simulink model "PACEWIPgbug2version13"  (R2022b)
settings: Solver=FixedStepAuto  StartTime=0.0  StopTime=10  FixedStep=1e-3  RelTol=1e-3  EnableMultiTasking=on
undefined symbols (not defined in the file): A0, A1, D0, D1, D10, D11, D12, D13, D2, D3, D4, D5, D6, D7, D8, D9, PTA0, PTA1, PTA2, PTB2, PTB23, PTB3, PTB9, PTC16, PTC17, PTC2, PTC3, PTC4, PTD0, PTD1, PTD2, PTD3
libraries: frdmk64flib x21
settings Model: PacingRate=0.400000  ExtModeTrigDuration=5  Creator=carlo  LastModifiedBy=skaad
settings OptimizationCC: EnhancedBackFolding=on  PassReuseOutputArgsThreshold=0  MaxStackSize=64  OptimizeBlockOrder=speed  DifferentSizesBufferReuse=on  OptimizationCustomize=off
settings DebuggingCC: ParameterTunabilityLossMsg=error  UnconnectedInputMsg=warning  UnconnectedOutputMsg=warning  UnconnectedLineMsg=warning
settings HardwareCC: ProdBitPerPointer=32  ProdBitPerSizeT=32  ProdBitPerPtrDiffT=32  ProdLargestAtomicInteger=Long  ProdLargestAtomicFloat=Double  ProdWordSize=32  ProdHWDeviceType=ARM Compatible->ARM Cortex  UseEmbeddedCoderFeatures=off
settings ModelReferenceCC: EnableRefExpFcnMdlSchedulingChecks=on
settings SFSimCC: MATLABDynamicMemAlloc=off
settings RTWCC: Description=Embedded Coder  SystemTargetFile=ert.tlc  HardwareBoard=NXP FRDM-K64F  TLCOptions="-aInlineSetEventsForThisBaseRateFcn=TLC_FALSE -aSuppressMultiTaskScheduler=TLC_FALSE  -aRateBasedStepFcn=0"  TemplateMakefile=ert_default_tmf  Toolchain=GNU Tools for ARM Embedded Processors  DLArmComputeVersion=19.05
settings CodeAppCC: ForceParamTrailComments=on  OperatorAnnotations=on
settings ERTTargetCC: ERTCustomFileBanners=off  SupportContinuousTime=on  SupportNonInlinedSFcns=on  RemoveResetFunc=off  ModelStepFunctionPrototypeControlCompliant=off  ExtModeTransport=4  ExtModeMexFile=sendToCommService

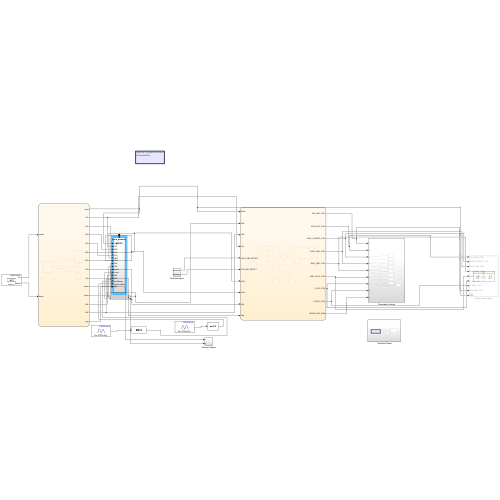
[thumbnail: Simulink's stored preview of the top-level diagram]
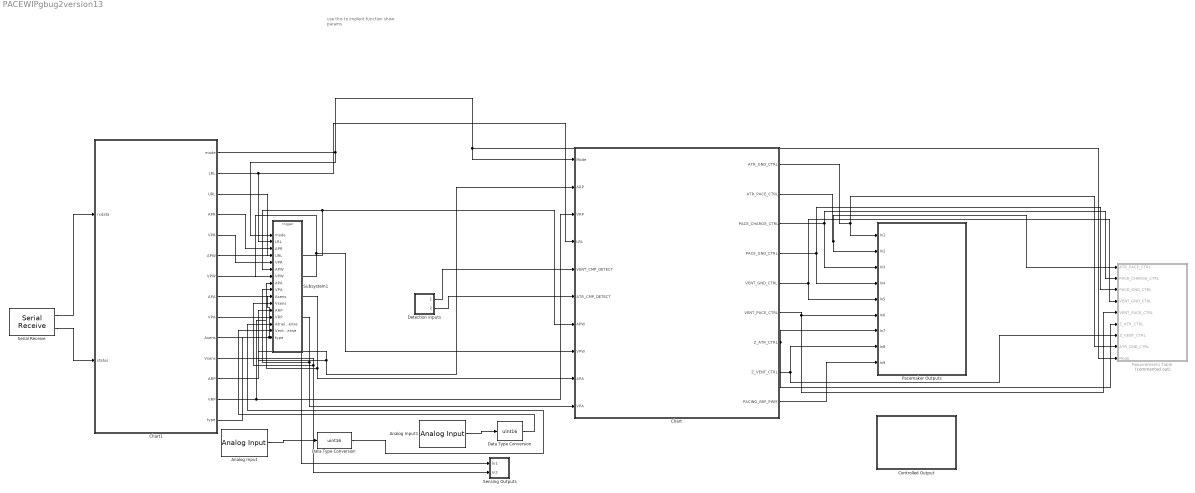
== system PACEWIPgbug2version13 ==
  note: use this to implent function
      | show params
  Analog Input : frdmk64flib/Analog Input  Whichpin=PTB2 (A0)  SampleTime=-1
  Analog Input1 : frdmk64flib/Analog Input  Whichpin=PTB3 (A1)  SampleTime=-1
  Chart : Stateflow chart  TreatAsAtomicUnit=on
  Chart1 : Stateflow chart  TreatAsAtomicUnit=on
  Controlled Output : Subsystem
  Data Type Conversion : DataTypeConversion  OutDataTypeStr=uint16  SaturateOnIntegerOverflow=off  RndMeth=Floor
  Data Type Conversion : DataTypeConversion  OutDataTypeStr=uint16  SaturateOnIntegerOverflow=off  RndMeth=Floor
  Detection inputs : Subsystem
  Pacemaker Outputs : Subsystem
  Requirements Table : Requirements Table  Commented=on  TreatAsAtomicUnit=on
  Sensing Outputs : Subsystem
  Serial Receive : frdmk64flib/Serial Receive  SCIModule=0  Baudrate=uint32(9600)  Parity=None  StopBits=1  HardwareFlowControl=None  ByteOrder=LittleEndian  DataType=uint8  DataLength=28  BlockingMode=off  OutputStatus=on  SampleTime=-1
  Subsystem1 : Subsystem
  wires:
  Chart/1(ATR_GND_CTRL) -> Requirements Table/8(ATR_GND_CTRL), Pacemaker Outputs/1(In1)
  Chart/2(ATR_PACE_CTRL) -> Requirements Table/1(ATR_PACE_CTRL), Pacemaker Outputs/2(In2)
  Chart/4(PACE_GND_CTRL) -> Pacemaker Outputs/4(In4), Requirements Table/3(PACE_GND_CTRL)
  Chart/5(VENT_GND_CTRL) -> Pacemaker Outputs/5(In5), Requirements Table/4(VENT_GND_CTRL)
  Chart/6(VENT_PACE_CTRL) -> Requirements Table/5(VENT_PACE_CTRL), Pacemaker Outputs/6(In6)
  Chart/7(Z_ATR_CTRL) -> Requirements Table/6(Z_ATR_CTRL), Pacemaker Outputs/7(In7)
  Chart/8(Z_VENT_CTRL) -> Requirements Table/7(Z_VENT_CTRL), Pacemaker Outputs/8(In8)
  Chart/9(PACING_REF_PWM) -> Pacemaker Outputs/9(In9)
  Chart/3(PACE_CHARGE_CTRL) -> Pacemaker Outputs/3(In3), Requirements Table/2(PACE_CHARGE_CTRL)
  Chart1/1(mode) -> Chart/1(Mode), Requirements Table/9(Mode), Subsystem1/1(mode)
  Chart1/12(ARP) -> Chart/2(ARP), Subsystem1/12(ARP)
  Chart1/13(VRP) -> Chart/3(VRP), Subsystem1/13(VRP)
  Chart1/2(LRL) -> Chart/4(LRL), Subsystem1/2(LRL)
  Chart1/6(APW) -> Chart/7(APW), Subsystem1/6(APW)
  Serial Receive/1 -> Chart1/1(rxdata)
  Chart1/3(URL) -> Subsystem1/4(URL)
  Chart1/4(APR) -> Subsystem1/3(APR)
  Chart1/5(VPR) -> Subsystem1/5(VPR)
  Chart1/7(VPW) -> Subsystem1/7(VPW), Chart/8(VPW)
  Chart1/8(APA) -> Subsystem1/8(APA), Chart/9(APA)
  Chart1/9(VPA) -> Subsystem1/9(VPA), Chart/10(VPA)
  Detection inputs/1(VentricularSense) -> Chart/5(VENT_CMP_DETECT)
  Detection inputs/2(AtrialSense) -> Chart/6(ATR_CMP_DETECT)
  Chart1/11(Vsens) -> Subsystem1/11(Vsens), Sensing Outputs/2(In2)
  Chart1/10(Asens) -> Sensing Outputs/1(In1), Subsystem1/10(Asens)
  Serial Receive/2 -> Chart1/2(status)
  Analog Input1/1 -> Data Type Conversion/1
  Data Type Conversion/1 -> Subsystem1/15(VentricularSense)
  Analog Input/1 -> Data Type Conversion/1
  Data Type Conversion/1 -> Subsystem1/14(AtrialSense)
  Chart1/14(type) -> Subsystem1/16(type)

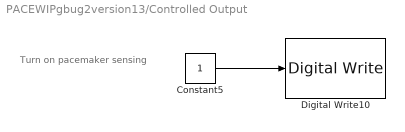
== system PACEWIPgbug2version13/Controlled Output ==
  note: Turn on pacemaker
      | sensing
  Constant5 : Constant
  Digital Write10 : frdmk64flib/Digital Write  Whichpin=PTD1 (D13)
  wires:
  Constant5/1 -> Digital Write10/1

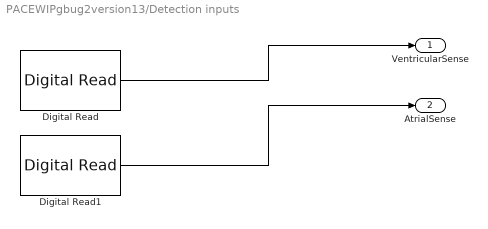
== system PACEWIPgbug2version13/Detection inputs ==
  Digital Read : frdmk64flib/Digital Read  Whichpin=PTC17 (D1)  SampleTime=-1
  Digital Read1 : frdmk64flib/Digital Read  Whichpin=PTC16 (D0)  SampleTime=-1
  VentricularSense : Outport
  AtrialSense : Outport  Port=2
  wires:
  Digital Read/1 -> VentricularSense/1
  Digital Read1/1 -> AtrialSense/1

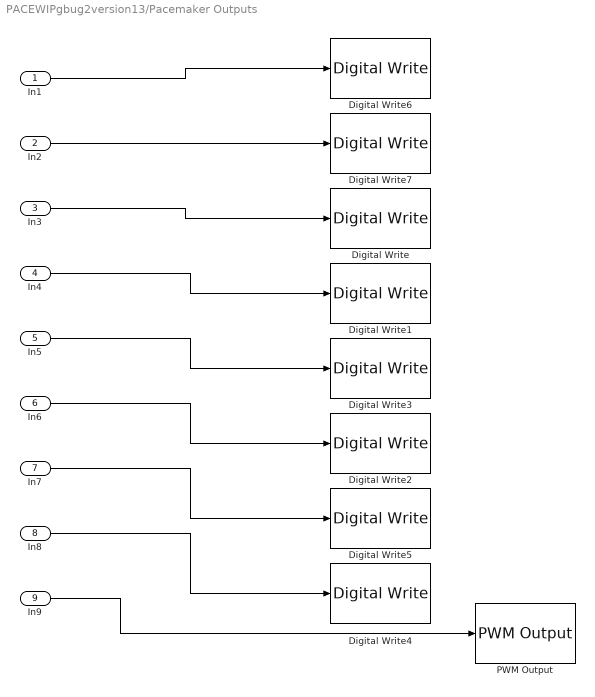
== system PACEWIPgbug2version13/Pacemaker Outputs ==
  In1 : Inport
  In2 : Inport  Port=2
  In3 : Inport  Port=3
  In4 : Inport  Port=4
  In5 : Inport  Port=5
  In6 : Inport  Port=6
  In7 : Inport  Port=7
  In8 : Inport  Port=8
  In9 : Inport  Port=9
  Digital Write : frdmk64flib/Digital Write  Whichpin=PTB9 (D2)
  Digital Write1 : frdmk64flib/Digital Write  Whichpin=PTD0 (D10)
  Digital Write2 : frdmk64flib/Digital Write  Whichpin=PTC4 (D9)
  Digital Write3 : frdmk64flib/Digital Write  Whichpin=PTD3 (D12)
  Digital Write4 : frdmk64flib/Digital Write  Whichpin=PTC3 (D7)
  Digital Write5 : frdmk64flib/Digital Write  Whichpin=PTB23 (D4)
  Digital Write6 : frdmk64flib/Digital Write  Whichpin=PTD2 (D11)
  Digital Write7 : frdmk64flib/Digital Write  Whichpin=PTA0 (D8)
  PWM Output : frdmk64flib/PWM Output  Whichpin=PTA2 (D5)  InitialFrequency=2000  InitialDutyCycle=60
  wires:
  In1/1 -> Digital Write6/1
  In3/1 -> Digital Write/1
  In2/1 -> Digital Write7/1
  In4/1 -> Digital Write1/1
  In9/1 -> PWM Output/1
  In7/1 -> Digital Write5/1
  In6/1 -> Digital Write2/1
  In8/1 -> Digital Write4/1
  In5/1 -> Digital Write3/1

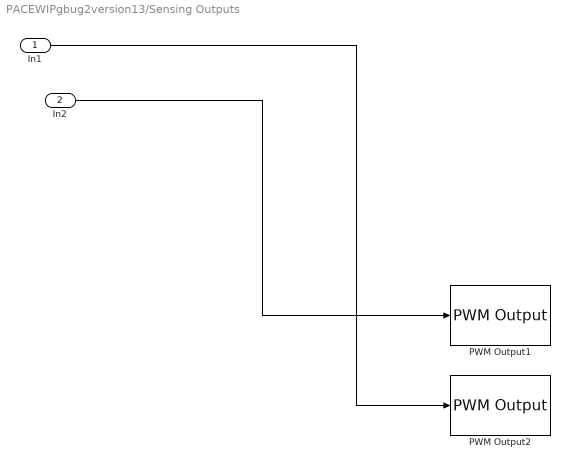
== system PACEWIPgbug2version13/Sensing Outputs ==
  In1 : Inport
  In2 : Inport  Port=2
  PWM Output1 : frdmk64flib/PWM Output  Whichpin=PTA1 (D3)  InitialFrequency=2000  InitialDutyCycle=60
  PWM Output2 : frdmk64flib/PWM Output  Whichpin=PTC2 (D6)  InitialFrequency=2000  InitialDutyCycle=60
  wires:
  In1/1 -> PWM Output2/1
  In2/1 -> PWM Output1/1

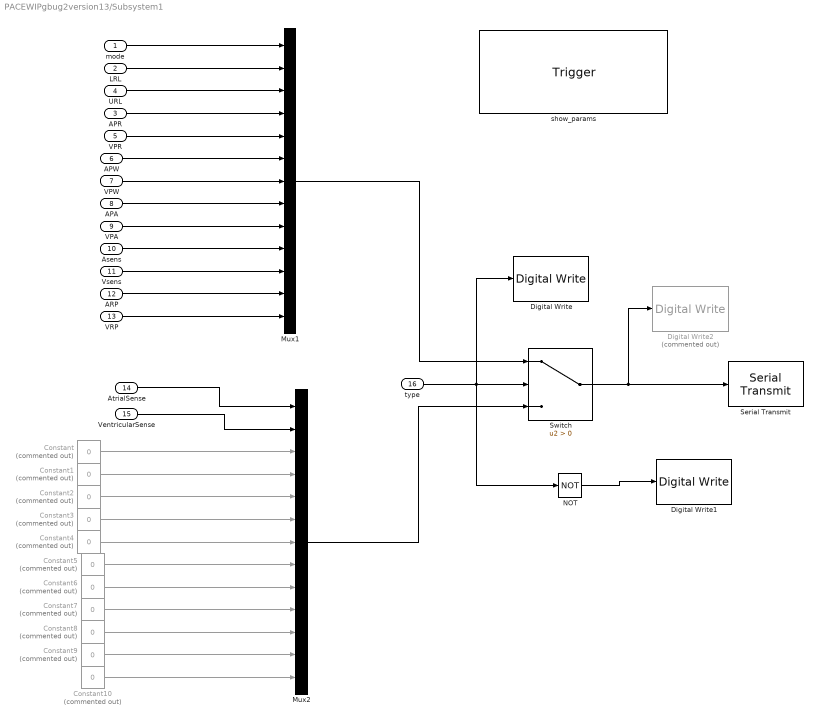
== system PACEWIPgbug2version13/Subsystem1 ==
  mode : Inport
  LRL : Inport  Port=2
  APR : Inport  Port=3
  URL : Inport  Port=4
  VPR : Inport  Port=5
  APW : Inport  Port=6
  VPW : Inport  Port=7
  APA : Inport  Port=8
  VPA : Inport  Port=9
  Asens : Inport  Port=10
  Vsens : Inport  Port=11
  ARP : Inport  Port=12
  VRP : Inport  Port=13
  AtrialSense : Inport  Port=14
  VentricularSense : Inport  Port=15
  type : Inport  Port=16
  show_params : TriggerPort  TriggerType=function-call  IsSimulinkFunction=on  FunctionName=show_params  VariantControl=(inherit)
  Constant{,1..10} (11 alike) : Constant  Commented=on  Value=0  OutDataTypeStr=uint16
  Digital Write : frdmk64flib/Digital Write  Whichpin=BLUE_LED
  Digital Write1 : frdmk64flib/Digital Write  Whichpin=RED_LED
  Digital Write2 : frdmk64flib/Digital Write  Commented=on  Whichpin=GREEN_LED
  Mux1 : Mux  Inputs=13
  Mux2 : Mux  Inputs=13
  NOT : Logic  Operator=NOT  IconShape=distinctive  AllPortsSameDT=off  OutDataTypeStr=boolean
  Serial Transmit : frdmk64flib/Serial Transmit  SCIModule=0  Baudrate=uint32(9600)  Parity=None  StopBits=1  HardwareFlowControl=None  ByteOrder=LittleEndian  BlockingMode=on  OutputStatus=off
  Switch : Switch  Criteria=u2 > Threshold  SaturateOnIntegerOverflow=off  InputSameDT=off
  wires:
  VPR/1 -> Mux1/5
  VPA/1 -> Mux1/9
  ARP/1 -> Mux1/12
  APA/1 -> Mux1/8
  mode/1 -> Mux1/1
  Asens/1 -> Mux1/10
  VPW/1 -> Mux1/7
  APR/1 -> Mux1/4
  LRL/1 -> Mux1/2
  VRP/1 -> Mux1/13
  Vsens/1 -> Mux1/11
  Mux1/1 -> Switch/1
  type/1 -> NOT/1, Digital Write/1, Switch/2
  APW/1 -> Mux1/6
  URL/1 -> Mux1/3
  Switch/1 -> Digital Write2/1, Serial Transmit/1
  Constant/1 -> Mux2/3
  Constant1/1 -> Mux2/4
  AtrialSense/1 -> Mux2/1
  VentricularSense/1 -> Mux2/2
  Constant2/1 -> Mux2/5
  Constant3/1 -> Mux2/6
  Constant6/1 -> Mux2/9
  Constant7/1 -> Mux2/10
  Constant5/1 -> Mux2/8
  Constant4/1 -> Mux2/7
  Constant8/1 -> Mux2/11
  Constant9/1 -> Mux2/12
  Constant10/1 -> Mux2/13
  Mux2/1 -> Switch/3
  NOT/1 -> Digital Write1/1

== stateflow chart PACEWIPgbug2version13/Requirements Table ==
  (default) -> (junction 1073746513)
  (junction 1073746513) -> (junction 1073746514) : {
      | % SF_REQ_REV_07
      | }
  (junction 1073746514) -> (junction 1073746516) : {
      | % HEADER_ASSIGNMENTS
      |
      | }
  (junction 1073746516) -> (junction 1073746518) : {
      | % START_A_4
      | }
  (junction 1073746518) -> (junction 1073746520) : {
      | }
  (junction 1073746520) -> (junction 1073746522)
  (junction 1073746522) -> (junction 1073746524) : {
      | }
  (junction 1073746524) -> (junction 1073746526) : {
      | % END_A_4
      | }
  (junction 1073746526) -> (junction 1073746528) : {
      | % START_R_1
      | }
  (junction 1073746528) -> (junction 1073746530) : {
      | }
  (junction 1073746530) -> (junction 1073746532) : {
      |
      |
      | }
  (junction 1073746532) -> (junction 1073746534) : {
      | }
  (junction 1073746534) -> (junction 1073746590) : {
      | % START_R_16
      | }
  (junction 1073746590) -> (junction 1073746592) : {
      | }
  (junction 1073746592) -> (junction 1073746594)
  (junction 1073746594) -> (junction 1073746596) [order 1] : [duration((Mode==1)) >= 1]
  (junction 1073746594) -> (junction 1073746602) [order 2]
  (junction 1073746596) -> (junction 1073746598) : {
      | reqtable_postcondition((((ATR_PACE_CTRL) == (0))) && (((VENT_PACE_CTRL) == (0))) && (((PACE_CHARGE_CTRL) == (1))) && (((PACE_GND_CTRL) == (0))) && (((ATR_GND_CTRL) == (1))) && (((VENT_GND_CTRL) == (0))) && (((Z_ATR_CTRL) == (0))) && (((Z_VENT_CTRL) == (0))), 'R:1.1');
      |
      |
      | }
  (junction 1073746598) -> (junction 1073746600) : {
      | }
  (junction 1073746600) -> (junction 1073746602)
  (junction 1073746602) -> (junction 1073746604)
  (junction 1073746604) -> (junction 1073746606) : {
      | % END_R_16
      | }
  (junction 1073746606) -> (junction 1073746611) : {
      | % START_R_22
      | }
  (junction 1073746611) -> (junction 1073746613) : {
      | }
  (junction 1073746613) -> (junction 1073746615)
  (junction 1073746615) -> (junction 1073746617) [order 1] : [duration((Mode==1)) >= 1]
  (junction 1073746615) -> (junction 1073746623) [order 2]
  (junction 1073746617) -> (junction 1073746619) : {
      | reqtable_postcondition((((ATR_PACE_CTRL) == (1))) && (((VENT_PACE_CTRL) == (0))) && (((PACE_CHARGE_CTRL) == (0))) && (((PACE_GND_CTRL) == (1))) && (((ATR_GND_CTRL) == (0))) && (((VENT_GND_CTRL) == (0))) && (((Z_ATR_CTRL) == (0))) && (((Z_VENT_CTRL) == (0))), 'R:1.2');
      |
      |
      | }
  (junction 1073746619) -> (junction 1073746621) : {
      | }
  (junction 1073746621) -> (junction 1073746623)
  (junction 1073746623) -> (junction 1073746625)
  (junction 1073746625) -> (junction 1073746627) : {
      | % END_R_22
      | }
  (junction 1073746627) -> (junction 1073746556) : {
      | % END_R_1
      | }
  (junction 1073746556) -> (junction 1073746674) : {
      | % START_R_7
      | }
  (junction 1073746674) -> (junction 1073746676) : {
      | }
  (junction 1073746676) -> (junction 1073746678) : {
      |
      |
      | }
  (junction 1073746678) -> (junction 1073746680) : {
      | }
  (junction 1073746680) -> (junction 1073746682) : {
      | % START_R_28
      | }
  (junction 1073746682) -> (junction 1073746684) : {
      | }
  (junction 1073746684) -> (junction 1073746686)
  (junction 1073746686) -> (junction 1073746688) [order 1] : [duration((Mode==2)) >= 1]
  (junction 1073746686) -> (junction 1073746694) [order 2]
  (junction 1073746688) -> (junction 1073746690) : {
      | reqtable_postcondition((((ATR_PACE_CTRL) == (0))) && (((VENT_PACE_CTRL) == (0))) && (((PACE_CHARGE_CTRL) == (1))) && (((PACE_GND_CTRL) == (0))) && (((ATR_GND_CTRL) == (0))) && (((VENT_GND_CTRL) == (1))) && (((Z_ATR_CTRL) == (0))) && (((Z_VENT_CTRL) == (0))), 'R:2.1');
      |
      |
      | }
  (junction 1073746690) -> (junction 1073746692) : {
      | }
  (junction 1073746692) -> (junction 1073746694)
  (junction 1073746694) -> (junction 1073746696)
  (junction 1073746696) -> (junction 1073746698) : {
      | % END_R_28
      | }
  (junction 1073746698) -> (junction 1073746700) : {
      | % START_R_31
      | }
  (junction 1073746700) -> (junction 1073746702) : {
      | }
  (junction 1073746702) -> (junction 1073746704)
  (junction 1073746704) -> (junction 1073746706) [order 1] : [duration((Mode==2)) >= 1]
  (junction 1073746704) -> (junction 1073746712) [order 2]
  (junction 1073746706) -> (junction 1073746708) : {
      | reqtable_postcondition((((ATR_PACE_CTRL) == (0))) && (((VENT_PACE_CTRL) == (1))) && (((PACE_CHARGE_CTRL) == (0))) && (((PACE_GND_CTRL) == (1))) && (((ATR_GND_CTRL) == (0))) && (((VENT_GND_CTRL) == (0))) && (((Z_ATR_CTRL) == (0))) && (((Z_VENT_CTRL) == (0))), 'R:2.2');
      |
      |
      | }
  (junction 1073746708) -> (junction 1073746710) : {
      | }
  (junction 1073746710) -> (junction 1073746712)
  (junction 1073746712) -> (junction 1073746714)
  (junction 1073746714) -> (junction 1073746716) : {
      | % END_R_31
      | }
  (junction 1073746716) -> (junction 1073746718) : {
      | % END_R_7
      | }
  (junction 1073746718) -> (junction 1073746724) : {
      | % START_R_10
      | }
  (junction 1073746724) -> (junction 1073746726) : {
      | }
  (junction 1073746726) -> (junction 1073746728) : {
      |
      |
      | }
  (junction 1073746728) -> (junction 1073746730) : {
      | }
  (junction 1073746730) -> (junction 1073746732) : {
      | % START_R_46
      | }
  (junction 1073746732) -> (junction 1073746734) : {
      | }
  (junction 1073746734) -> (junction 1073746736)
  (junction 1073746736) -> (junction 1073746738) [order 1] : [duration((Mode==3)) >= 1]
  (junction 1073746736) -> (junction 1073746744) [order 2]
  (junction 1073746738) -> (junction 1073746740) : {
      | reqtable_postcondition((((ATR_PACE_CTRL) == (0))) && (((VENT_PACE_CTRL) == (0))) && (((PACE_CHARGE_CTRL) == (1))) && (((PACE_GND_CTRL) == (0))) && (((ATR_GND_CTRL) == (1))) && (((VENT_GND_CTRL) == (0))) && (((Z_ATR_CTRL) == (0))) && (((Z_VENT_CTRL) == (0))), 'R:3.1');
      |
      |
      | }
  (junction 1073746740) -> (junction 1073746742) : {
      | }
  (junction 1073746742) -> (junction 1073746744)
  (junction 1073746744) -> (junction 1073746746)
  (junction 1073746746) -> (junction 1073746748) : {
      | % END_R_46
      | }
  (junction 1073746748) -> (junction 1073746750) : {
      | % START_R_61
      | }
  (junction 1073746750) -> (junction 1073746752) : {
      | }
  (junction 1073746752) -> (junction 1073746754)
  (junction 1073746754) -> (junction 1073746756) [order 1] : [duration((Mode==3)) >= 1]
  (junction 1073746754) -> (junction 1073746762) [order 2]
  (junction 1073746756) -> (junction 1073746758) : {
      | reqtable_postcondition((((ATR_PACE_CTRL) == (1))) && (((VENT_PACE_CTRL) == (0))) && (((PACE_CHARGE_CTRL) == (0))) && (((PACE_GND_CTRL) == (1))) && (((ATR_GND_CTRL) == (0))) && (((VENT_GND_CTRL) == (0))) && (((Z_ATR_CTRL) == (0))) && (((Z_VENT_CTRL) == (0))), 'R:3.2');
      |
      |
      | }
  (junction 1073746758) -> (junction 1073746760) : {
      | }
  (junction 1073746760) -> (junction 1073746762)
  (junction 1073746762) -> (junction 1073746764)
  (junction 1073746764) -> (junction 1073746766) : {
      | % END_R_61
      | }
  (junction 1073746766) -> (junction 1073746768) : {
      | % END_R_10
      | }
  (junction 1073746768) -> (junction 1073746774) : {
      | % START_R_13
      | }
  (junction 1073746774) -> (junction 1073746776) : {
      | }
  (junction 1073746776) -> (junction 1073746778) : {
      |
      |
      | }
  (junction 1073746778) -> (junction 1073746780) : {
      | }
  (junction 1073746780) -> (junction 1073746782) : {
      | % START_R_49
      | }
  (junction 1073746782) -> (junction 1073746784) : {
      | }
  (junction 1073746784) -> (junction 1073746786)
  (junction 1073746786) -> (junction 1073746788) [order 1] : [duration((Mode==4)) >= 1]
  (junction 1073746786) -> (junction 1073746794) [order 2]
  (junction 1073746788) -> (junction 1073746790) : {
      | reqtable_postcondition((((ATR_PACE_CTRL) == (0))) && (((VENT_PACE_CTRL) == (0))) && (((PACE_CHARGE_CTRL) == (1))) && (((PACE_GND_CTRL) == (0))) && (((ATR_GND_CTRL) == (0))) && (((VENT_GND_CTRL) == (1))) && (((Z_ATR_CTRL) == (0))) && (((Z_VENT_CTRL) == (0))), 'R:4.1');
      |
      |
      | }
  (junction 1073746790) -> (junction 1073746792) : {
      | }
  (junction 1073746792) -> (junction 1073746794)
  (junction 1073746794) -> (junction 1073746796)
  (junction 1073746796) -> (junction 1073746798) : {
      | % END_R_49
      | }
  (junction 1073746798) -> (junction 1073746800) : {
      | % START_R_58
      | }
  (junction 1073746800) -> (junction 1073746802) : {
      | }
  (junction 1073746802) -> (junction 1073746804)
  (junction 1073746804) -> (junction 1073746806) [order 1] : [duration((Mode==4)) >= 1]
  (junction 1073746804) -> (junction 1073746812) [order 2]
  (junction 1073746806) -> (junction 1073746808) : {
      | reqtable_postcondition((((ATR_PACE_CTRL) == (0))) && (((VENT_PACE_CTRL) == (1))) && (((PACE_CHARGE_CTRL) == (0))) && (((PACE_GND_CTRL) == (1))) && (((ATR_GND_CTRL) == (0))) && (((VENT_GND_CTRL) == (0))) && (((Z_ATR_CTRL) == (0))) && (((Z_VENT_CTRL) == (0))), 'R:4.2');
      |
      |
      | }
  (junction 1073746808) -> (junction 1073746810) : {
      | }
  (junction 1073746810) -> (junction 1073746812)
  (junction 1073746812) -> (junction 1073746814)
  (junction 1073746814) -> (junction 1073746816) : {
      | % END_R_58
      | }
  (junction 1073746816) -> (junction 1073746818) : {
      | % END_R_13
      | }
  data: ATR_PACE_CTRL input double; PACE_CHARGE_CTRL input; PACE_GND_CTRL input; VENT_GND_CTRL input; VENT_PACE_CTRL input; Z_ATR_CTRL input; Z_VENT_CTRL input; ATR_GND_CTRL input; Mode input

== stateflow chart PACEWIPgbug2version13/Chart ==
  state AOO_PACE
    entry:
    PACE_CHARGE_CTRL=0;
    PACE_GND_CTRL=1;
    VENT_PACE_CTRL=0
    VENT_GND_CTRL=0;
    Z_ATR_CTRL=0;
    Z_VENT_CTRL=0;
    ATR_GND_CTRL=0;
    ATR_PACE_CTRL=1
  state AOO_CHARGE
    entry:
    ATR_PACE_CTRL=0;
    VENT_PACE_CTRL=0;
    PACING_REF_PWM=APA;
    PACE_CHARGE_CTRL=1;
    PACE_GND_CTRL=1;
    Z_ATR_CTRL=0;
    Z_VENT_CTRL=0;
    VENT_GND_CTRL=0;
    ATR_GND_CTRL=1
  state VVI_CHARGE
    ATR_PACE_CTRL=0;
    VENT_PACE_CTRL=0;
    PACING_REF_PWM=VPA;
    PACE_CHARGE_CTRL=1;
    PACE_GND_CTRL=1;
    Z_ATR_CTRL=0;
    Z_VENT_CTRL=0;
    ATR_GND_CTRL=0;
    VENT_GND_CTRL=1
  state VVI_Refractory
  state MODE_SELECT
  state VOO_CHARGE
    entry:
    ATR_PACE_CTRL=0;
    VENT_PACE_CTRL=0;
    PACING_REF_PWM=VPA;
    PACE_CHARGE_CTRL=1;
    PACE_GND_CTRL=1;
    Z_ATR_CTRL=0;
    Z_VENT_CTRL=0;
    ATR_GND_CTRL=0;
    VENT_GND_CTRL=1
  state VOO_PACE
    entry:
    PACE_CHARGE_CTRL=0;
    PACE_GND_CTRL=1;
    ATR_PACE_CTRL=0
    ATR_GND_CTRL=0;
    Z_ATR_CTRL=0;
    Z_VENT_CTRL=0;
    VENT_GND_CTRL=0;
    VENT_PACE_CTRL=1
  state VVI_SENSING
  state VVI_PACE
    entry:
    PACE_CHARGE_CTRL=0;
    PACE_GND_CTRL=1;
    ATR_PACE_CTRL=0
    ATR_GND_CTRL=0;
    Z_ATR_CTRL=0;
    Z_VENT_CTRL=0;
    VENT_GND_CTRL=0;
    VENT_PACE_CTRL=1
  state AAI_CHARGE
    entry:
    ATR_PACE_CTRL = 0;
    VENT_PACE_CTRL = 0;
    PACING_REF_PWM = APA;
    PACE_CHARGE_CTRL = 1;
    PACE_GND_CTRL = 1;
    Z_ATR_CTRL = 0;
    Z_VENT_CTRL = 0;
    VENT_GND_CTRL = 0;
    ATR_GND_CTRL = 1
  state AAI_Refractory
  state AAI_SENSING
  state AAI_PACE
    entry:
    PACE_CHARGE_CTRL = 0;
    PACE_GND_CTRL = 1;
    VENT_PACE_CTRL = 0;
    VENT_GND_CTRL = 0;
    Z_ATR_CTRL = 0;
    Z_VENT_CTRL = 0;
    ATR_GND_CTRL = 0;
    ATR_PACE_CTRL = 1
  MODE_SELECT -> VVI_CHARGE [order 3] : [Mode==4]
  VVI_CHARGE -> MODE_SELECT [order 1] : [Mode~=4]
  AOO_CHARGE -> AOO_PACE [order 1] : after(1000-APW,msec)
  AOO_PACE -> AOO_CHARGE : after(APW,msec)
  MODE_SELECT -> AOO_CHARGE [order 2] : [Mode == 1]
  VVI_PACE -> VVI_CHARGE : after(VPW,msec)
  (default) -> MODE_SELECT
  VVI_CHARGE -> VVI_Refractory [order 2] : after(1,msec)
  AOO_CHARGE -> MODE_SELECT [order 2] : [Mode~=1]
  VVI_SENSING -> VVI_Refractory [order 2] : [VENT_CMP_DETECT == 1]
  MODE_SELECT -> VOO_CHARGE [order 1] : [Mode == 2]
  VVI_Refractory -> VVI_SENSING : after(VRP,msec)
  VOO_CHARGE -> MODE_SELECT [order 2] : [Mode~=2]
  MODE_SELECT -> AAI_CHARGE [order 4] : [Mode==3]
  AAI_CHARGE -> MODE_SELECT [order 1] : [Mode~=3]
  VOO_CHARGE -> VOO_PACE [order 1] : after(1000-VPW,msec)
  VOO_PACE -> VOO_CHARGE : after(VPW,msec)
  VVI_SENSING -> VVI_PACE [order 1] : after(60000/LRL-VRP,msec)
  AAI_PACE -> AAI_CHARGE : after(APW,msec)
  AAI_CHARGE -> AAI_Refractory [order 2] : after(1,msec)
  AAI_SENSING -> AAI_Refractory [order 2] : [ATR_CMP_DETECT == 1]
  AAI_Refractory -> AAI_SENSING : after(ARP,msec)
  AAI_SENSING -> AAI_PACE [order 1] : after(60000/LRL-ARP,msec)
  data: ATR_GND_CTRL output; ATR_PACE_CTRL output; PACE_CHARGE_CTRL output; PACE_GND_CTRL output; VENT_GND_CTRL output; VENT_PACE_CTRL output; Z_ATR_CTRL output; Z_VENT_CTRL output; Mode input; PACING_REF_PWM output; ARP input; VRP input; LRL input; VENT_CMP_DETECT input; ATR_CMP_DETECT input; APW input; VPW input; APA input; VPA input

== stateflow chart PACEWIPgbug2version13/Chart1 ==
  settings: executeAtInitialization=1
  state set_param
    % setting parameters
    entry:
    type=1;
    mode=typecast(rxdata(3:4), 'uint16');
    LRL=typecast(rxdata(5:6), 'uint16');
    URL=typecast(rxdata(7:8), 'uint16');
    APR=typecast(rxdata(9:10), 'uint16');
    VPR=typecast(rxdata(11:12), 'uint16');
    APW=typecast(rxdata(13:14), 'uint16');
    VPW=typecast(rxdata(15:16), 'uint16');
    APA=typecast(rxdata(17:18), 'uint16');
    VPA=typecast(rxdata(19:20), 'uint16');
    Asens=typecast(rxdata(21:22), 'uint16');
    Vsens=typecast(rxdata(23:24), 'uint16');
    ARP=typecast(rxdata(25:26), 'uint16');
    VRP=typecast(rxdata(27:28), 'uint16');
    show_params();
    %rxdata(15)=0;
  state Initial
    % entry state
    entry:
    type=0
    mode=0;
    LRL=0;
    URL=0;
    APR=0;
    VPR=0;
    APW=0;
    VPW=0;
    APA=0;
    VPA=0;
    Asens=0;
    Vsens=0;
    ARP=0;
    VRP=0;
  state Standby_
    % waits for stattus to change
  state Echo
    %if asked
    entry:
    show_params();
  state send_ecg
    % showing param
    entry:
    type=0;
    show_params();
  set_param -> Standby_
  (default) -> Initial
  (junction 58) -> set_param [order 1] : [rxdata(2)==hex2dec('55')]
  (junction 58) -> Echo [order 3] : [rxdata(2)==hex2dec('47')]
  Initial -> Standby_
  Standby_ -> (junction 47) : [status==0]
  (junction 47) -> (junction 58) : [rxdata(1)==hex2dec('16')]
  (junction 58) -> send_ecg [order 2] : [rxdata(2)==hex2dec('49')]
  Echo -> Standby_
  send_ecg -> Standby_
  data: rxdata input uint8; status input uint8; mode output uint16; LRL output uint16; URL output uint16; APR output uint16; VPR output uint16; APW output uint16; VPW output uint16; APA output uint16; VPA output uint16; Asens output uint16; Vsens output uint16; ARP output uint16; VRP output uint16; type output
